simulink model "RLCLow_verify"  (R2022b)
settings: Solver=VariableStepAuto  StartTime=0.0  StopTime=0.001  RelTol=1e-3
InitFcn:
  | rng("shuffle");
  | %seed = round(rand(1)*1000);
  | seed = 100;
StopFcn:
  | writematrix(out.input, "C:\Users\dmesenge\Documents\School\PattRecNN\Project\models\RLCLow_test_inputs.csv")
  | writematrix(out.actual, "C:\Users\dmesenge\Documents\School\PattRecNN\Project\models\RLCLow_test_outputs.csv")
libraries: fl_lib x5, nesl_utility x3, simulink x2, ee_lib x1
settings Model: Creator=dmesenge  LastModifiedBy=dmesenge

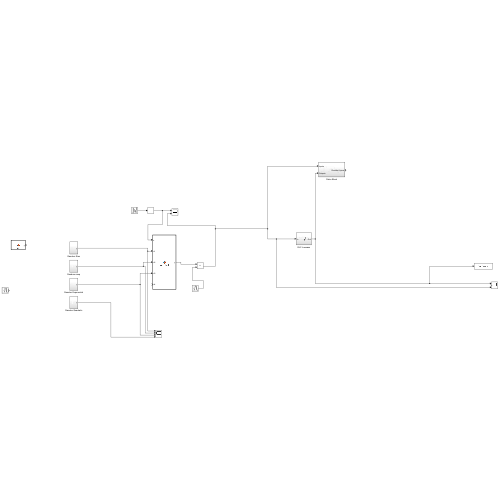
[thumbnail: Simulink's stored preview of the top-level diagram]
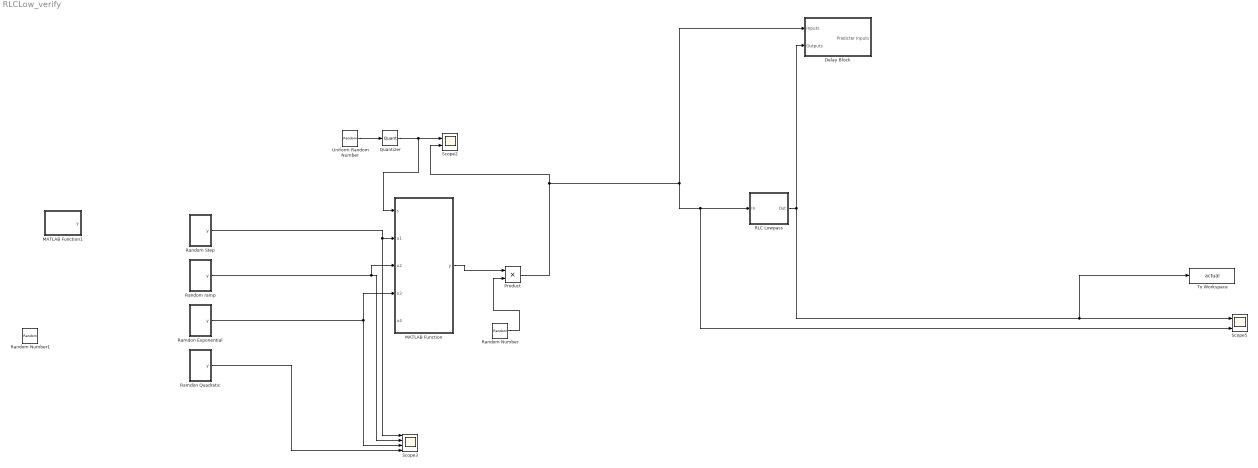
== system RLCLow_verify ==
  Delay Block : Subsystem
  MATLAB Function : MATLAB Function  TreatAsAtomicUnit=on
  MATLAB Function1 : MATLAB Function  TreatAsAtomicUnit=on
  Product : Product
  Quantizer : Quantizer  QuantizationInterval=1
  RLC Lowpass : Subsystem
  Ramdon Exponential : Subsystem
  Ramdon Quadratic : Subsystem
  Random Number : RandomNumber  SampleTime=0.0001
  Random Number1 : RandomNumber  SampleTime=0.00000001
  Random Step : Subsystem
  Random ramp : Subsystem
  Scope2 : Scope  NumInputPorts=2
  Scope3 : Scope  NumInputPorts=4
  Scope5 : Scope  NumInputPorts=3
  To Workspace : ToWorkspace  VariableName=actual  SampleTime=-1
  Uniform Random Number : UniformRandomNumber  Minimum=1  Maximum=4  SampleTime=0.00001
  wires:
  Quantizer/1 -> MATLAB Function/1(s), Scope2/1
  Ramdon Quadratic/1(y) -> Scope3/4
  Random Number/1 -> Product/2
  Random Step/1(y) -> Scope3/1, MATLAB Function/2(u1)
  Ramdon Exponential/1(y) -> Scope3/3, MATLAB Function/4(u3)
  MATLAB Function/1(y) -> Product/1
  Random ramp/1(y) -> MATLAB Function/3(u2), Scope3/2
  Uniform Random Number/1 -> Quantizer/1
  Product/1 -> Delay Block/1(Inputs), RLC Lowpass/1(In), Scope5/3, Scope2/2
  RLC Lowpass/1(Out) -> Delay Block/2(Outputs), To Workspace/1, Scope5/1

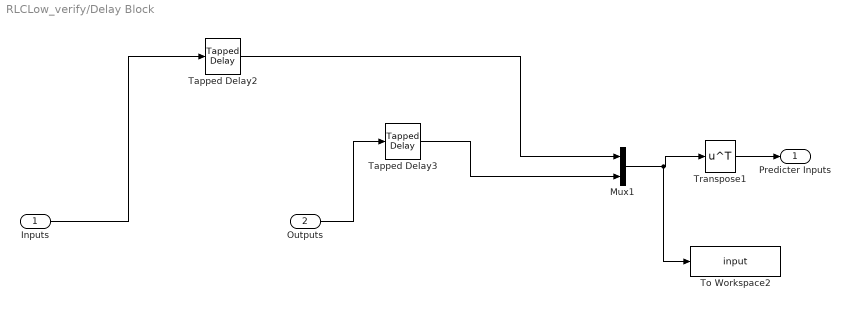
== system RLCLow_verify/Delay Block ==
  Inputs : Inport
  Outputs : Inport  Port=2
  Mux1 : Mux  Inputs=2
  Tapped Delay2 : simulink/Discrete/Tapped Delay  vinit=0.0  samptime=-1  NumDelays=9  DelayOrder=Newest  includeCurrent=on
  Tapped Delay3 : simulink/Discrete/Tapped Delay  vinit=0.0  samptime=-1  NumDelays=9  DelayOrder=Newest  includeCurrent=on
  To Workspace2 : ToWorkspace  VariableName=input  SampleTime=-1
  Transpose1 : Math  Operator=transpose
  Predicter Inputs : Outport
  wires:
  Mux1/1 -> To Workspace2/1, Transpose1/1
  Tapped Delay2/1 -> Mux1/1
  Inputs/1 -> Tapped Delay2/1
  Tapped Delay3/1 -> Mux1/2
  Outputs/1 -> Tapped Delay3/1
  Transpose1/1 -> Predicter Inputs/1

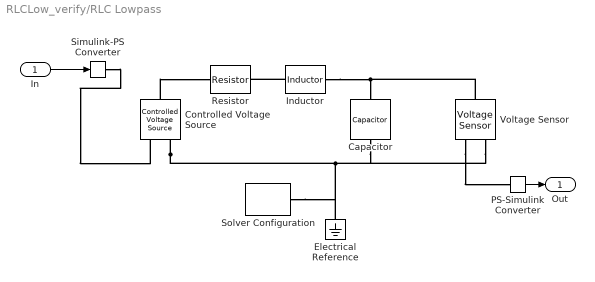
== system RLCLow_verify/RLC Lowpass ==
  In : Inport
  Capacitor : fl_lib/Electrical/Electrical Elements/Capacitor  c=1e-6 F  r=1e-6 Ohm  g=0 1/Ohm  i_specify=off  i_priority=None  i=0 A  i_nominal_specify=off  i_nominal_unit=A  i_nominal_value=1  v_specify=off  v_priority=None  v=0 V  v_nominal_specify=off  v_nominal_unit=V  v_nominal_value=1  vc_specify=off  vc_priority=High  vc=0 V  vc_nominal_specify=off  vc_nominal_unit=V  vc_nominal_value=1
  Controlled Voltage Source : fl_lib/Electrical/Electrical Sources/Controlled Voltage Source
  Electrical Reference : fl_lib/Electrical/Electrical Elements/Electrical Reference
  Inductor : fl_lib/Electrical/Electrical Elements/Inductor  l=1e-6 H  r=0 Ohm  g=1e-9 1/Ohm  i_specify=off  i_priority=None  i=0 A  i_nominal_specify=off  i_nominal_unit=A  i_nominal_value=1  v_specify=off  v_priority=None  v=0 V  v_nominal_specify=off  v_nominal_unit=V  v_nominal_value=1  i_L_specify=off  i_L_priority=High  i_L=0 A  i_L_nominal_specify=off  i_L_nominal_unit=A  i_L_nominal_value=1
  PS-Simulink Converter : nesl_utility/PS-Simulink Converter  PhysicalDomain=network_engine_domain  SubClassName=ps_output  LeftPortType=input  RightPortType=output  PseudoPeriodic=off  Frequencies=[]  VectorFormat=inherit  Unit=inherit  AffineConversion=off
  Resistor : ee_lib/Passive/Resistor  R=10 Ohm  enable_R_tol=0  R_tol=5  tol_distribution=1  nSigma=4  enable_operating_limits=0  operating_limit_action=2  max_working_voltage=100 V  power_rating=1 W  enable_faults=0  fault_action=1  R_faulted=inf Ohm  enable_temporal_fault=0  t_fault=1 s  enable_behavioral_fault=0  max_permissible_current=1 A  t_fail_on_current=1 s  noise_mode=0  sample_time=1e-3 s  repeatability=1  auto_seed=664334928  user_seed=0  Tdevice=25 degC  power_derating_T1=70 degC  power_derating_T2=155 degC  operating_temperature_range_vec=[-50, 150] degC  alpha=3.93e-3 1/K  Tmeas=25 degC  thermal_mass=100 J/K  temperature_specify=off  temperature_priority=High  temperature=298.15 K  temperature_nominal_specify=off  temperature_nominal_unit=K  temperature_nominal_value=1
  Simulink-PS Converter : nesl_utility/Simulink-PS Converter  PhysicalDomain=network_engine_domain  SubClassName=ps_input  LeftPortType=input  RightPortType=output  PseudoPeriodic=off  Frequencies=[]  NoiseDistribution=none  NoiseParameters=[]  Unit=1  AffineConversion=off  FilteringAndDerivatives=provide  SimscapeFilterOrder=1  InputFilterTimeConstant=0.001  UdotUserProvided=0
  Solver Configuration : nesl_utility/Solver Configuration  PhysicalDomain=network_engine_domain  SubClassName=solver  LeftPortType=input  RightPortType=generic  Tones=[]  Harmonics=[]  SimulateNoise=off  Profile=off  UseLocalSampling=off  EnableSwitchedLinearOptims=on  FrequencyDomain=off  UseCCode=off  RelTol=0.001  AbsTol=0.001  MinStep=1e-09  ToWorkspace=off  RevertToSquareIcSolve=off  NumHomotopyIterations=100  PhasorMode=off  PhasorModeNumHarmonics=1  ConsistencySolver=NEWTON_XTOL_AFTER_FTOL  IndexReductionMethod=DerivativeReplacement  DoDC=off  ResidualTolerance=1e-09  ConsistencyTolSource=GLOBAL  ConsistencyAbsTol=0.001  ConsistencyRelTol=0.001  ConsistencyTolFactor=0.001  UseLocalSolver=off  LocalSolverChoice=NE_BACKWARD_EULER_ADVANCER  ResolveIndetEquations=on  FunctionEvalNumThread=1  LocalSolverSampleTime=0.001  DoFixedCost=off  MaxNonlinIter=3  MaxModeIter=2  ComputeImpulses=off  ImpulseIterations=2  LinearAlgebra=auto  LinearAlgebraNumThread=0  EquationFormulation=NE_TIME_EF  DelaysMemoryBudget=1024  AutomaticFiltering=on  FilteringTimeConstant=0.001  PartitionStorageMethod=AS_NEEDED  PartitionMemoryBudget=1024  PartitionMethod=ROBUST
  Voltage Sensor : fl_lib/Electrical/Electrical Sensors/Voltage Sensor
  Out : Outport
  wires:
  In/1 -> Simulink-PS Converter/1
  PS-Simulink Converter/1 -> Out/1
  connections:
  Controlled Voltage Source/RConn2 -- Capacitor/RConn1 -- Voltage Sensor/RConn2 -- Solver Configuration/RConn1 -- Electrical Reference/LConn1
  Controlled Voltage Source/LConn1 -- Resistor/LConn1
  Voltage Sensor/RConn1 -- PS-Simulink Converter/LConn1
  Simulink-PS Converter/RConn1 -- Controlled Voltage Source/RConn1
  Voltage Sensor/LConn1 -- Inductor/RConn1 -- Capacitor/LConn1
  Inductor/LConn1 -- Resistor/RConn1

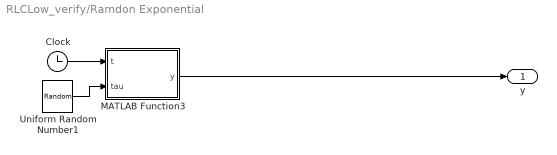
== system RLCLow_verify/Ramdon Exponential ==
  Clock : Clock
  MATLAB Function3 : MATLAB Function  TreatAsAtomicUnit=on
  Uniform Random Number1 : UniformRandomNumber  Minimum=-1000  Maximum=1000  Seed=seed  SampleTime=0.00001
  y : Outport
  wires:
  Clock/1 -> MATLAB Function3/1(t)
  Uniform Random Number1/1 -> MATLAB Function3/2(tau)
  MATLAB Function3/1(y) -> y/1

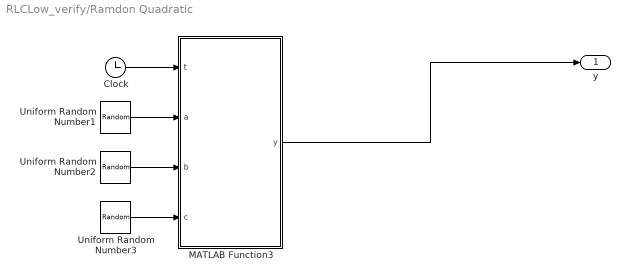
== system RLCLow_verify/Ramdon Quadratic ==
  Clock : Clock
  MATLAB Function3 : MATLAB Function  TreatAsAtomicUnit=on
  Uniform Random Number1 : UniformRandomNumber  Minimum=-10  Maximum=10  Seed=seed  SampleTime=0.00001
  Uniform Random Number2 : UniformRandomNumber  Minimum=-100  Maximum=100  Seed=seed  SampleTime=0.00001
  Uniform Random Number3 : UniformRandomNumber  Minimum=-1000  Maximum=1000  Seed=seed  SampleTime=0.00001
  y : Outport
  wires:
  Clock/1 -> MATLAB Function3/1(t)
  Uniform Random Number1/1 -> MATLAB Function3/2(a)
  MATLAB Function3/1(y) -> y/1
  Uniform Random Number3/1 -> MATLAB Function3/4(c)
  Uniform Random Number2/1 -> MATLAB Function3/3(b)

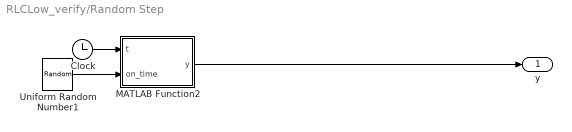
== system RLCLow_verify/Random Step ==
  Clock : Clock
  MATLAB Function2 : MATLAB Function  TreatAsAtomicUnit=on
  Uniform Random Number1 : UniformRandomNumber  Minimum=0  Maximum=0.001  Seed=seed  SampleTime=0.00001
  y : Outport
  wires:
  Uniform Random Number1/1 -> MATLAB Function2/2(on_time)
  Clock/1 -> MATLAB Function2/1(t)
  MATLAB Function2/1(y) -> y/1

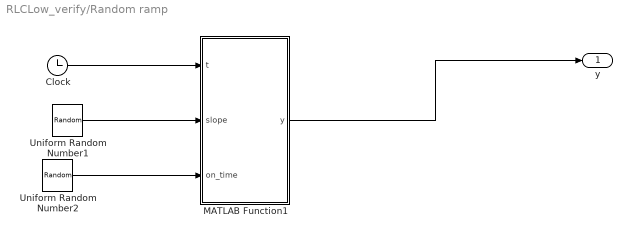
== system RLCLow_verify/Random ramp ==
  Clock : Clock
  MATLAB Function1 : MATLAB Function  TreatAsAtomicUnit=on
  Uniform Random Number1 : UniformRandomNumber  Minimum=-10000  Maximum=10000  Seed=seed  SampleTime=0.00001
  Uniform Random Number2 : UniformRandomNumber  Minimum=0  Maximum=0.001  Seed=seed  SampleTime=0.00001
  y : Outport
  wires:
  Uniform Random Number2/1 -> MATLAB Function1/3(on_time)
  Clock/1 -> MATLAB Function1/1(t)
  Uniform Random Number1/1 -> MATLAB Function1/2(slope)
  MATLAB Function1/1(y) -> y/1

== matlab function RLCLow_verify/Random ramp/MATLAB Function1 ==
  settings: updateMethod=DISCRETE
  data: t input; y output; slope input; on_time input
function y = rand_ramp(t, slope, on_time)
    %random slope
%     min = -100;
%     max = 100;
%     slope = min+rand()*(max-min);
% 
%     %random on time
%     min = 0;
%     max = 0.001;
%     on_time = min+rand()*(max-min);

    if t < on_time
        r = 0;
    else
        r = slope*t;
    end

y = r;

== matlab function RLCLow_verify/MATLAB Function ==
  data: s input; u1 input; y output; u2 input; u3 input; u4 input
function y = mux_4to1(s, u1, u2, u3, u4)
    switch s
       case 1
          r = u1;
       case 2
          r = u2;
       case 3
          r = u3;
       case 4
          r = u4;
       otherwise
          r = u1;
    end

y = r;

== matlab function RLCLow_verify/Random Step/MATLAB Function2 ==
  settings: updateMethod=DISCRETE
  data: t input; y output; on_time input
function y = rand_step(t, on_time)

    %random on time
%     min = 0;
%     max = 0.001;
%     on_time = min+rand()*(max-min);

    if t < on_time
        r = 0;
    else
        r = 1;
    end

y = r;

== matlab function RLCLow_verify/Ramdon Exponential/MATLAB Function3 ==
  settings: updateMethod=DISCRETE
  data: t input; y output; tau input
function y = rand_exp(t, tau)
    r = exp(t*tau);

y = r;

== matlab function RLCLow_verify/Ramdon Quadratic/MATLAB Function3 ==
  settings: updateMethod=DISCRETE
  data: t input; y output; a input; b input; c input
function y = rand_exp(t, a, b, c)
    r = a*t*t + b*t + c;

y = r;

== matlab function RLCLow_verify/MATLAB Function1 ==
  data: y output
function y = fcn()
seed = rand(1);
y = rand(1);
